simulink model "tether2node_th"  (R2018b)
settings: Solver=VariableStepAuto  StartTime=0.0  StopTime=10.0  RelTol=1e-3
values from neighbouring files (symbols this model uses):
  flow = [0;0;0]    [tether2node_ts.m]
  numTethers = 3    [tether2node_ts.m]
libraries: tether2node_ul x1
settings Model: Creator=asiddiq2  LastModifiedBy=asiddiq2

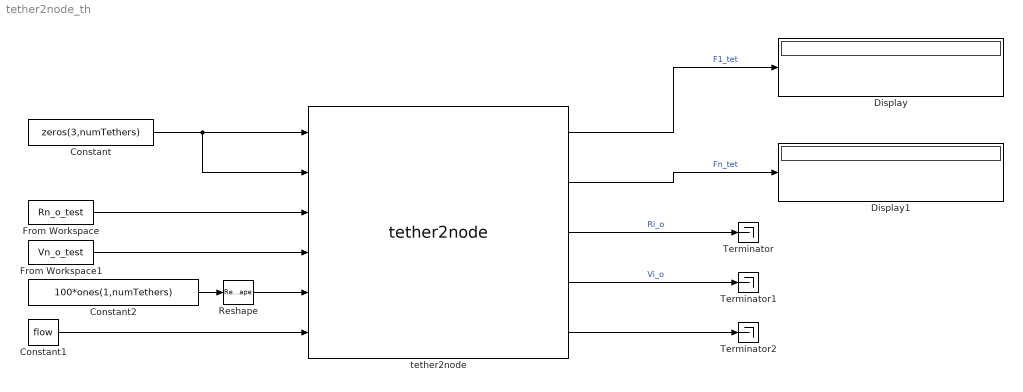
== system tether2node_th ==
  Constant : Constant  Value=zeros(3,numTethers)  VectorParams1D=off
  Constant1 : Constant  Value=flow  VectorParams1D=off
  Constant2 : Constant  Value=100*ones(1,numTethers)  VectorParams1D=off
  Display : Display
  Display1 : Display
  From Workspace : FromWorkspace  VariableName=Rn_o_test  SampleTime=0
  From Workspace1 : FromWorkspace  VariableName=Vn_o_test  SampleTime=0
  Reshape : Reshape  OutputDimensionality=Row vector (2-D)
  Terminator : Terminator
  Terminator1 : Terminator
  Terminator2 : Terminator
  tether2node : tether2node_ul/tether2node  rhoFluid=rho_fluid  massBdy=mass  numNode=thr.numNodes.Value  thrDia=thr.thrDiameter.Value  thrRho=thr.thrDensity.Value  thrYoungs=thr.thrYoungs.Value  thrZeta=thr.thrDampingRatio.Value  thrCd=thr.thrDragCoeff.Value
  wires:
  From Workspace/1 -> tether2node/3
  From Workspace1/1 -> tether2node/4
  Reshape/1 -> tether2node/5
  Constant/1 -> tether2node/2, tether2node/1
  Constant2/1 -> Reshape/1
  Constant1/1 -> tether2node/6
  tether2node/5 -> Terminator2/1
  tether2node/2 -> Display1/1  "Fn_tet"
  tether2node/3 -> Terminator/1  "Ri_o"
  tether2node/4 -> Terminator1/1  "Vi_o"
  tether2node/1 -> Display/1  "F1_tet"
